simulink model "db4_8znzrb"  (R2018a)
settings: Solver=ode23s  StartTime=0.0  StopTime=0.45  MaxStep=1e-3  RelTol=1e-4  AbsTol=1e-3
values from neighbouring files (symbols this model uses):
  Ian = 5    [set_motor.m]
  Kn = 0.6    [set_motor.m]
libraries: simulink x2
settings Model: ExtModeTrigMode=oneshot  ExtModeArmWhenConnect=off  Creator=Lac User  LastModifiedBy=Matias
settings SolverCC: AutoScaleAbsTol=off  MaxOrder=1  ZeroCrossAlgorithm=Adaptive
settings DataIOCC: LimitDataPoints=on  SaveFormat=Array  SignalLoggingSaveFormat=ModelDataLogs  SaveOutput=off  SaveTime=off
settings OptimizationCC: BlockReduction=off  BooleanDataType=off  LifeSpan=inf
settings DebuggingCC: SaveWithParameterizedLinksMsg=none  UnderspecifiedInitializationDetection=Classic  MergeDetectMultiDrivingBlocksExec=none  SignalResolutionControl=TryResolveAllWithWarning  MultiTaskDSMMsg=warning  MultiTaskCondExecSysMsg=none  SFUnexpectedBacktrackingDiag=warning  SFNoUnconditionalDefaultTransitionDiag=warning  SFExecutionAtInitializationDiag=none
settings HardwareCC: ProdBitPerPointer=32  ProdBitPerSizeT=32  ProdBitPerPtrDiffT=32  ProdLargestAtomicFloat=None  ProdIntDivRoundTo=Undefined  ProdEndianess=Unspecified  ProdWordSize=32  ProdHWDeviceType=32-bit Generic  TargetUnknown=on
settings ModelReferenceCC: PropagateSignalLabelsOutOfModel=off
settings RTWCC: TemplateMakefile=grt_vc.tmf
settings CodeAppCC: StateflowObjectComments=on
settings GRTTargetCC: TargetLangStandard=C89/C90 (ANSI)  GeneratePreprocessorConditionals=Disable all  CombineOutputUpdateFcns=off  GRTInterface=on
settings ConfigComp: CovMetricSettings=dw  CovHtmlReporting=on  CovSaveCumulativeToWorkspaceVar=on  CovSaveSingleToWorkspaceVar=on  CovExternalEMLEnable=off

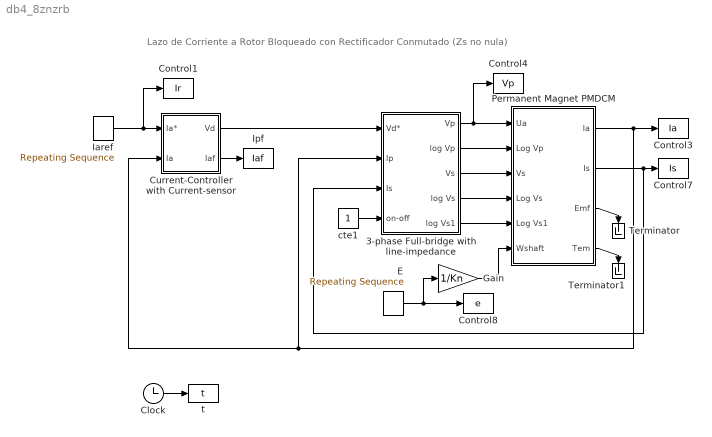
== system db4_8znzrb ==
  note: Lazo de Corriente a Rotor Bloqueado con Rectificador Conmutado (Zs no nula)
  3-phase Full-bridge with line-impedance : Subsystem  mask(3-phase Full-bridge with line-impedance){Vph=220, f=50, Rd=0.05, Ld=0.003, Rs=0.006, Ls=0.0002}
      mask prompts: Vph "RMS Phase Voltage [V]:"; f "Frecuency [Hz]:"; Rd "Armature Resistance [Ohms]:"; Ld "Armature Inductance  [Hy]:"; Rs "Line Resistance [Ohms]:"; Ls "Line Inductance [Hy]:"
  Clock : Clock
  Control1 : ToWorkspace  VariableName=Ir
      settings: MaxDataPoints=200000
  Control3 : ToWorkspace  VariableName=Ia
      settings: MaxDataPoints=200000
  Control4 : ToWorkspace  VariableName=Vp
      settings: MaxDataPoints=200000
  Control7 : ToWorkspace  VariableName=Is
      settings: MaxDataPoints=200000
  Control8 : ToWorkspace  VariableName=e
      settings: MaxDataPoints=200000
  Current-Controller with Current-sensor : Subsystem  mask(Current-Controller with Current-sensor){Kpi=0.16, TIi=0.027, Kti=1, Tfi=0.008, VLL=380}
      mask prompts: Kpi "Current Proportional Gain:"; TIi "Current Integral Gain:"; Kti "Current-sensor Proportional Gain:"; Tfi "Current-sensor Integral Gain:"; VLL "RMS Line to Line Voltage [V]:"
  E : simulink/Sources/Repeating Sequence  rep_seq_t="[0   0.4]"  rep_seq_y="[10   10 ]"
  Gain : Gain  Gain=1/Kn  SaturateOnIntegerOverflow=on  OutDataTypeStr=Inherit: Same as input  ParamDataTypeStr=Inherit: Same as input
  Iaref : simulink/Sources/Repeating Sequence  rep_seq_t=[0 0.4]  rep_seq_y=[Ian Ian]
  Ipf : ToWorkspace  VariableName=Iaf
      settings: MaxDataPoints=200000
  Permanent Magnet PMDCM : Subsystem  mask(Permanent Magnet PMDCM){La=0.003, Ra=0.05, k=6.7851, ic=0, Ls=0.0002, Rs=0.006}
      mask prompts: La "Armature Inductance  [Hy]:"; Ra "Armature Resistance [Ohms]:"; k "Motor Constant:"; ic "Armature Current Initial Condition [Amp]:"; Ls "Line Inductance [Hy]:"; Rs "Line Resistance [Ohms]:"
  Terminator : Terminator
  Terminator1 : Terminator
  cte1 : Constant
  t : ToWorkspace  VariableName=t
      settings: MaxDataPoints=200000
  wires:
  Iaref/1 -> Control1/1, Current-Controller with Current-sensor/1(Ia*)
  Current-Controller with Current-sensor/2(Iaf) -> Ipf/1
  E/1 -> Control8/1, Gain/1
  cte1/1 -> 3-phase Full-bridge with line-impedance/4(on-off)
  Current-Controller with Current-sensor/1(Vd) -> 3-phase Full-bridge with line-impedance/1(Vd*)
  3-phase Full-bridge with line-impedance/1(Vp) -> Control4/1, Permanent Magnet PMDCM/1(Ua)
  Gain/1 -> Permanent Magnet PMDCM/6(Wshaft)
  3-phase Full-bridge with line-impedance/2(log Vp) -> Permanent Magnet PMDCM/2(Log Vp)
  3-phase Full-bridge with line-impedance/3(Vs) -> Permanent Magnet PMDCM/3(Vs)
  3-phase Full-bridge with line-impedance/4(log Vs) -> Permanent Magnet PMDCM/4(Log Vs)
  3-phase Full-bridge with line-impedance/5(log Vs1) -> Permanent Magnet PMDCM/5(Log Vs1)
  Permanent Magnet PMDCM/1(Ia) -> Control3/1, Current-Controller with Current-sensor/2(Ia), 3-phase Full-bridge with line-impedance/2(Ip)
  Permanent Magnet PMDCM/2(Is) -> 3-phase Full-bridge with line-impedance/3(Is), Control7/1
  Permanent Magnet PMDCM/3(Emf) -> Terminator/1
  Permanent Magnet PMDCM/4(Tem) -> Terminator1/1
  Clock/1 -> t/1

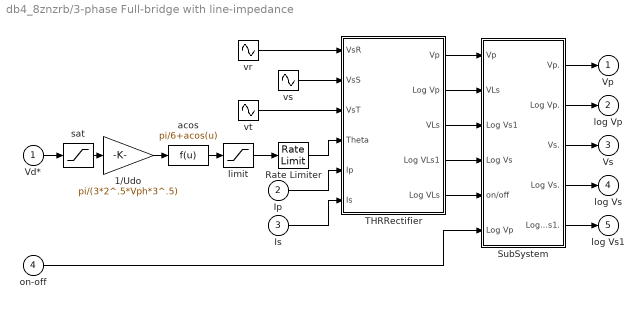
== system db4_8znzrb/3-phase Full-bridge with line-impedance ==
  Vd* : Inport
  Ip : Inport  Port=2
  Is : Inport  Port=3
  on-off : Inport  Port=4
  1/Udo : Gain  Gain=pi/(3*2^.5*Vph*3^.5)  SaturateOnIntegerOverflow=on  OutDataTypeStr=Inherit: Same as input  ParamDataTypeStr=Inherit: Same as input
  Rate Limiter : RateLimiter  RisingSlewLimit=8000  FallingSlewLimit=-8000
  SubSystem : Subsystem
  THRRectifier : Subsystem
      mask Display:
      | plot([0.3 0.7 0.5 0.3],[0.4 0.4 0.6 0.4])
      | plot([0.3 0.7 ],[0.6 0.6])
      | plot([0.5 0.5 ],[0.6 0.7])
      | plot([0.5 0.5 ],[0.3 0.4])
      | plot([0.35 0.5],[0.7 0.6])
      | plot([0.25 0.35 ],[0.7 0.7])
  acos : Fcn  Expr=pi/6+acos(u)
  limit : Saturate  UpperLimit=pi*6.999/6  LowerLimit=pi/5.998
  sat : Saturate  UpperLimit=(3*2^.5*3^.5*Vph)/pi  LowerLimit=-(3*2^.5*3^.5*Vph)/pi
  vr : Sin  Amplitude=Vph*(2^.5)  Frequency=2*f*pi  SampleTime=0
  vs : Sin  Amplitude=Vph*(2^.5)  Frequency=2*pi*f  Phase=-(2/3)*pi  SampleTime=0
  vt : Sin  Amplitude=Vph*(2^.5)  Frequency=2*pi*f  Phase=-(4/3)*pi  SampleTime=0
  Vp : Outport
  log Vp : Outport  Port=2
  Vs : Outport  Port=3
  log Vs : Outport  Port=4
  log Vs1 : Outport  Port=5
  wires:
  1/Udo/1 -> acos/1
  acos/1 -> limit/1
  vt/1 -> THRRectifier/3(VsT)
  vs/1 -> THRRectifier/2(VsS)
  vr/1 -> THRRectifier/1(VsR)
  Vd*/1 -> sat/1
  Ip/1 -> THRRectifier/5(Ip)
  Is/1 -> THRRectifier/6(Is)
  sat/1 -> 1/Udo/1
  limit/1 -> Rate Limiter/1
  THRRectifier/1(Vp) -> SubSystem/1(Vp)
  THRRectifier/2(Log Vp) -> SubSystem/2(VLs)
  THRRectifier/3(VLs) -> SubSystem/3(Log Vs1)
  THRRectifier/4(Log VLs1) -> SubSystem/4(Log Vs)
  THRRectifier/5(Log VLs) -> SubSystem/5(on/off)
  on-off/1 -> SubSystem/6(Log Vp)
  SubSystem/2(Log Vp.) -> log Vp/1
  SubSystem/3(Vs.) -> Vs/1
  SubSystem/4(Log Vs.) -> log Vs/1
  SubSystem/5(Log Vs1.) -> log Vs1/1
  SubSystem/1(Vp.) -> Vp/1
  Rate Limiter/1 -> THRRectifier/4(Theta)

== system db4_8znzrb/Current-Controller with Current-sensor ==
  Ia* : Inport
  Ia : Inport  Port=2
  Ftr : TransferFcn  Numerator=[Kti]  Denominator=[Tfi 1]
  I - Ctr : Subsystem
      mask Display: plot([0 .01  5],[0 2 4])
  Sum1 : Sum  Inputs=+-  SaturateOnIntegerOverflow=on  InputSameDT=on  OutDataTypeStr=Inherit: Same as first input
  Vd : Outport
  Iaf : Outport  Port=2
  wires:
  Ia*/1 -> Sum1/1
  Ia/1 -> Ftr/1, I - Ctr/2(Ia)
  Sum1/1 -> I - Ctr/1(Ia*- Iaf)
  I - Ctr/1(Vd*) -> Vd/1
  Ftr/1 -> Sum1/2, Iaf/1

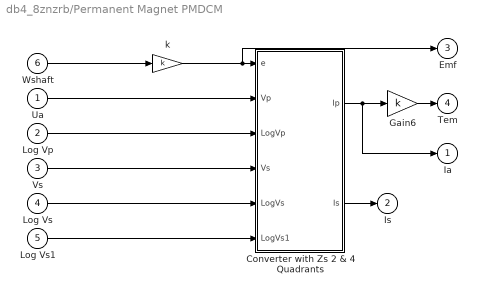
== system db4_8znzrb/Permanent Magnet PMDCM ==
  Ua : Inport
  Log Vp : Inport  Port=2
  Vs : Inport  Port=3
  Log Vs : Inport  Port=4
  Log Vs1 : Inport  Port=5
  Wshaft : Inport  Port=6
  Converter with Zs 2 & 4 Quadrants : Subsystem
  Gain6 : Gain  Gain=k  SaturateOnIntegerOverflow=on  OutDataTypeStr=Inherit: Same as input  ParamDataTypeStr=Inherit: Same as input
  k : Gain  Gain=k  SaturateOnIntegerOverflow=on  OutDataTypeStr=Inherit: Same as input  ParamDataTypeStr=Inherit: Same as input
  Ia : Outport
  Is : Outport  Port=2
  Emf : Outport  Port=3
  Tem : Outport  Port=4
  wires:
  k/1 -> Converter with Zs 2 & 4 Quadrants/1(e), Emf/1
  Ua/1 -> Converter with Zs 2 & 4 Quadrants/2(Vp)
  Log Vp/1 -> Converter with Zs 2 & 4 Quadrants/3(LogVp)
  Vs/1 -> Converter with Zs 2 & 4 Quadrants/4(Vs)
  Log Vs/1 -> Converter with Zs 2 & 4 Quadrants/5(LogVs)
  Log Vs1/1 -> Converter with Zs 2 & 4 Quadrants/6(LogVs1)
  Wshaft/1 -> k/1
  Converter with Zs 2 & 4 Quadrants/2(Is) -> Is/1
  Gain6/1 -> Tem/1
  Converter with Zs 2 & 4 Quadrants/1(Ip) -> Ia/1, Gain6/1

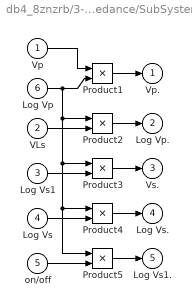
== system db4_8znzrb/3-phase Full-bridge with line-impedance/SubSystem ==
  Vp : Inport
  VLs : Inport  Port=2
  Log Vs1 : Inport  Port=3
  Log Vs : Inport  Port=4
  on/off : Inport  Port=5
  Log Vp : Inport  Port=6
  Product{1..5} (5 alike) : Product  SaturateOnIntegerOverflow=on  RndMeth=Zero  InputSameDT=on  OutDataTypeStr=Inherit: Same as first input
  Vp. : Outport
  Log Vp. : Outport  Port=2
  Vs. : Outport  Port=3
  Log Vs. : Outport  Port=4
  Log Vs1. : Outport  Port=5
  wires:
  VLs/1 -> Product2/2
  Log Vp/1 -> Product1/2, Product2/1, Product5/1, Product4/1, Product3/1
  Product2/1 -> Log Vp./1
  Product1/1 -> Vp./1
  Vp/1 -> Product1/1
  Log Vs1/1 -> Product3/2
  Log Vs/1 -> Product4/2
  on/off/1 -> Product5/2
  Product5/1 -> Log Vs1./1
  Product4/1 -> Log Vs./1
  Product3/1 -> Vs./1

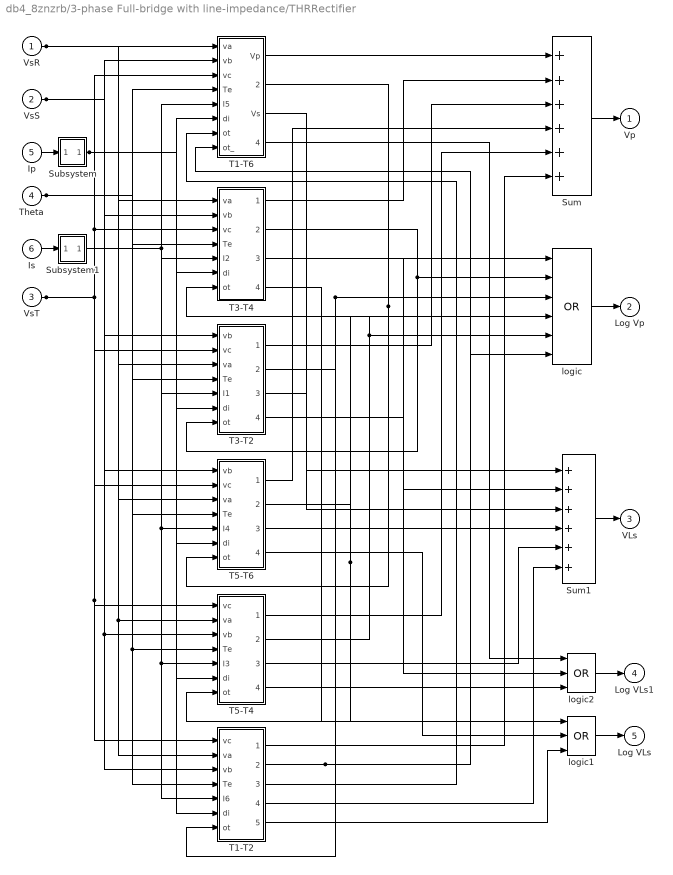
== system db4_8znzrb/3-phase Full-bridge with line-impedance/THRRectifier ==
  VsR : Inport
  VsS : Inport  Port=2
  VsT : Inport  Port=3
  Theta : Inport  Port=4
  Ip : Inport  Port=5
  Is : Inport  Port=6
  Subsystem : Subsystem
  Subsystem1 : Subsystem
  Sum : Sum  Inputs=++++++  SaturateOnIntegerOverflow=on  InputSameDT=on  OutDataTypeStr=Inherit: Same as first input
  Sum1 : Sum  Inputs=++++++  SaturateOnIntegerOverflow=on  InputSameDT=on  OutDataTypeStr=Inherit: Same as first input
  T1-T2 : Subsystem
  T1-T6 : Subsystem
  T3-T2 : Subsystem
  T3-T4 : Subsystem
  T5-T4 : Subsystem
  T5-T6 : Subsystem
  logic : Logic  Operator=OR  Inputs=6
  logic1 : Logic  Operator=OR  Inputs=3
  logic2 : Logic  Operator=OR  Inputs=3
  Vp : Outport
  Log Vp : Outport  Port=2
  VLs : Outport  Port=3
  Log VLs1 : Outport  Port=4
  Log VLs : Outport  Port=5
  wires:
  logic2/1 -> Log VLs1/1
  logic1/1 -> Log VLs/1
  Subsystem1/1(out_1) -> T1-T6/5(I5), T1-T2/5(I6), T5-T4/5(I3), T5-T6/5(I4), T3-T4/5(I2), T3-T2/5(I1)
  Subsystem/1(out_1) -> T5-T4/6(di), T5-T6/6(di), T3-T2/6(di), T3-T4/6(di), T1-T6/6(di), T1-T2/6(di)
  Theta/1 -> T1-T2/4(Te), T5-T4/4(Te), T5-T6/4(Te), T3-T2/4(Te), T3-T4/4(Te), T1-T6/4(Te)
  T1-T2/2(out_1) -> T1-T6/8(ot_), logic/6
  logic/1 -> Log Vp/1
  Sum/1 -> Vp/1
  Ip/1 -> Subsystem/1(in_1)
  Sum1/1 -> VLs/1
  T1-T6/2(Log Vp) -> T5-T6/7(ot), logic/1
  T1-T6/1(Vp) -> Sum/1
  T1-T6/3(Vs) -> Sum1/1
  T1-T6/4(Log Vs) -> logic2/1
  T3-T4/1(out_2) -> Sum/2
  VsR/1 -> T1-T6/1(va), T3-T4/1(va), T3-T2/3(va), T5-T6/3(va), T5-T4/2(va), T1-T2/2(va)
  VsS/1 -> T1-T6/2(vb), T3-T4/2(vb), T3-T2/1(vb), T5-T6/1(vb), T5-T4/3(vb), T1-T2/3(vb)
  T3-T4/2(out_1) -> T3-T2/7(ot), logic/2
  T3-T4/3(out_3) -> Sum1/2
  T3-T4/4(out_4) -> logic1/1
  T3-T2/1(out_2) -> Sum/3
  T3-T2/2(out_1) -> logic/3, T1-T2/7(ot)
  T3-T2/3(out_3) -> Sum1/3
  T3-T2/4(out_4) -> logic2/2
  VsT/1 -> T3-T2/2(vc), T1-T6/3(vc), T3-T4/3(vc), T5-T6/2(vc), T5-T4/1(vc), T1-T2/1(vc)
  T5-T6/2(out_1) -> T5-T4/7(ot), logic/4
  T5-T6/3(out_3) -> Sum1/4
  T5-T6/4(out_4) -> logic1/2
  T5-T6/1(out_2) -> Sum/4
  T5-T4/2(out_1) -> T3-T4/7(ot), logic/5
  T5-T4/1(out_2) -> Sum/5
  T5-T4/3(out_3) -> Sum1/5
  T5-T4/4(out_4) -> logic2/3
  T1-T2/3(out_3) -> T1-T6/7(ot)
  T1-T2/4("out_4 ") -> Sum1/6
  T1-T2/5(out_5) -> logic1/3
  T1-T2/1(out_2) -> Sum/6
  Is/1 -> Subsystem1/1(in_1)

== system db4_8znzrb/Current-Controller with Current-sensor/I - Ctr ==
  Ia*- Iaf : Inport
  Ia : Inport  Port=2
  Adaptative Control : Subsystem
  comp : RelationalOperator  Operator=>  RndMeth=Nearest  InputSameDT=on
  cte1 : Constant  Value=0
  sat : Saturate  UpperLimit=VLL*sqrt(2)*3/pi  LowerLimit=-VLL*sqrt(2)*3/pi
  Vd* : Outport
  wires:
  Ia*- Iaf/1 -> Adaptative Control/2(Ia*- Iaf)
  cte1/1 -> comp/2
  sat/1 -> Vd*/1
  Adaptative Control/1(Vd*) -> sat/1
  comp/1 -> Adaptative Control/1(Ia>0)
  Ia/1 -> comp/1

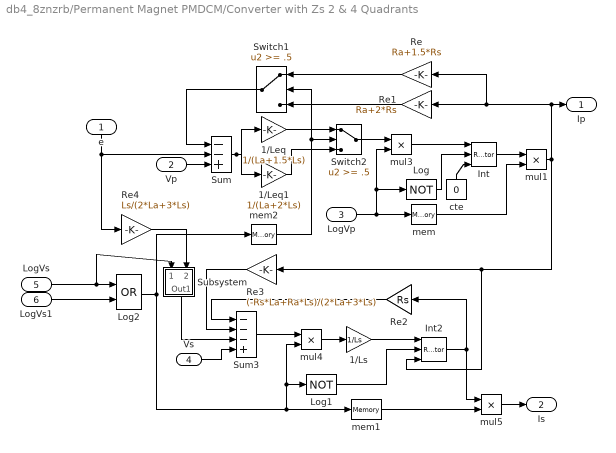
== system db4_8znzrb/Permanent Magnet PMDCM/Converter with Zs 2 & 4 Quadrants ==
  e : Inport
  Vp : Inport  Port=2
  LogVp : Inport  Port=3
  Vs : Inport  Port=4
  LogVs : Inport  Port=5
  LogVs1 : Inport  Port=6
  "1/Leq " : Gain  Gain=1/(La+1.5*Ls)  SaturateOnIntegerOverflow=on  OutDataTypeStr=Inherit: Same as input  ParamDataTypeStr=Inherit: Same as input
  1/Leq1 : Gain  Gain=1/(La+2*Ls)  SaturateOnIntegerOverflow=on  OutDataTypeStr=Inherit: Same as input  ParamDataTypeStr=Inherit: Same as input
  1/Ls : Gain  Gain=1/Ls  SaturateOnIntegerOverflow=on  OutDataTypeStr=Inherit: Same as input  ParamDataTypeStr=Inherit: Same as input
  Int : ResetIntegrator
  Int2 : ResetIntegrator
  Log : Logic  Operator=NOT  Inputs=1
  Log1 : Logic  Operator=NOT  Inputs=1
  Log2 : Logic  Operator=OR
  Re : Gain  Gain=Ra+1.5*Rs  SaturateOnIntegerOverflow=on  OutDataTypeStr=Inherit: Same as input  ParamDataTypeStr=Inherit: Same as input
  Re1 : Gain  Gain=Ra+2*Rs  SaturateOnIntegerOverflow=on  OutDataTypeStr=Inherit: Same as input  ParamDataTypeStr=Inherit: Same as input
  Re2 : Gain  Gain=Rs  SaturateOnIntegerOverflow=on  OutDataTypeStr=Inherit: Same as input  ParamDataTypeStr=Inherit: Same as input
  Re3 : Gain  Gain=(-Rs*La+Ra*Ls)/(2*La+3*Ls)  SaturateOnIntegerOverflow=on  OutDataTypeStr=Inherit: Same as input  ParamDataTypeStr=Inherit: Same as input
  Re4 : Gain  Gain=Ls/(2*La+3*Ls)  SaturateOnIntegerOverflow=on  OutDataTypeStr=Inherit: Same as input  ParamDataTypeStr=Inherit: Same as input
  Subsystem : Subsystem
      mask Display: disp('-1')
  Sum : Sum  Inputs=--+  SaturateOnIntegerOverflow=on  InputSameDT=on  OutDataTypeStr=Inherit: Same as first input
  Sum3 : Sum  Inputs=---+  SaturateOnIntegerOverflow=on  InputSameDT=on  OutDataTypeStr=Inherit: Same as first input
  Switch1 : Switch  Threshold=.5  SaturateOnIntegerOverflow=on  InputSameDT=on
  Switch2 : Switch  Threshold=.5  SaturateOnIntegerOverflow=on  InputSameDT=on
  cte : Constant  Value=0
  mem : Memory
  mem1 : Memory
  mem2 : Memory
  mul{1,3..5} (4 alike) : Product  SaturateOnIntegerOverflow=on  RndMeth=Zero  InputSameDT=on  OutDataTypeStr=Inherit: Same as first input
  Ip : Outport
  Is : Outport  Port=2
  wires:
  mem/1 -> mul1/2
  Int/1 -> mul1/1
  mul3/1 -> Int/1
  Log/1 -> Int/2
  cte/1 -> Int/3
  mul1/1 -> Re3/1, Int2/3, Ip/1, Re1/1, Re/1
  LogVp/1 -> mem/1, mul3/2, Log/1
  Switch2/1 -> mul3/1
  1/Leq1/1 -> Switch2/3
  "1/Leq "/1 -> Switch2/1
  Re/1 -> Switch1/1
  Re1/1 -> Switch1/3
  Vp/1 -> Sum/3
  mem2/1 -> Switch1/2, Switch2/2
  Sum/1 -> 1/Leq1/1, "1/Leq "/1
  Re3/1 -> Sum3/2
  Switch1/1 -> Sum/1
  LogVs/1 -> Subsystem/1(In1), Log2/1
  Vs/1 -> Sum3/4
  mul5/1 -> Is/1
  Re4/1 -> Subsystem/2(In2)
  Log2/1 -> mem2/1, mul4/2, Log1/1, mem1/1
  1/Ls/1 -> Int2/1
  mul4/1 -> 1/Ls/1
  Log1/1 -> Int2/2
  Re2/1 -> Sum3/1
  Sum3/1 -> mul4/1
  mem1/1 -> mul5/2
  Int2/1 -> Re2/1, mul5/1
  e/1 -> Sum/2, Re4/1
  Subsystem/1(Out1) -> Sum3/3
  LogVs1/1 -> Log2/2

== system db4_8znzrb/3-phase Full-bridge with line-impedance/THRRectifier/Subsystem ==
  in_1 : Inport
  comp : RelationalOperator  Operator=>  RndMeth=Nearest  InputSameDT=on
  cte : Constant  Value=0
  out_1 : Outport
  wires:
  cte/1 -> comp/2
  in_1/1 -> comp/1
  comp/1 -> out_1/1

== system db4_8znzrb/3-phase Full-bridge with line-impedance/THRRectifier/Subsystem1 ==
  in_1 : Inport
  Vdset : Step  Time=0  Before=1  SampleTime=0
  comp : RelationalOperator  Operator=>  RndMeth=Nearest  InputSameDT=on
  cte : Constant  Value=0
  mul : Product  SaturateOnIntegerOverflow=on  RndMeth=Zero  InputSameDT=on  OutDataTypeStr=Inherit: Same as first input
  out_1 : Outport
  wires:
  Vdset/1 -> mul/2
  mul/1 -> out_1/1
  comp/1 -> mul/1
  cte/1 -> comp/2
  in_1/1 -> comp/1

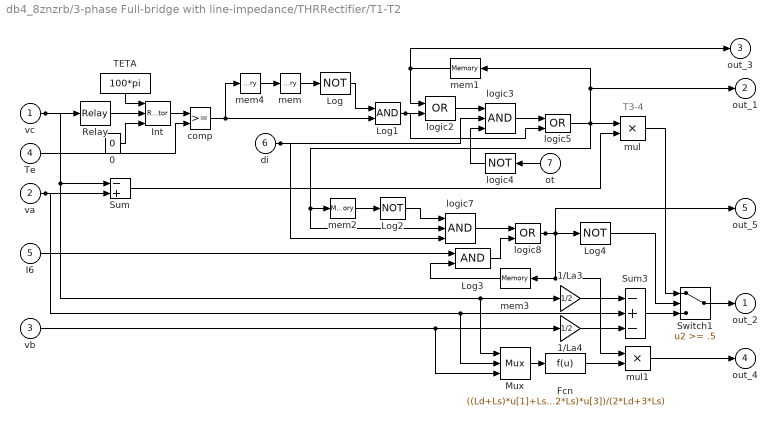
== system db4_8znzrb/3-phase Full-bridge with line-impedance/THRRectifier/T1-T2 ==
  note: T3-4
  vc : Inport
  va : Inport  Port=2
  vb : Inport  Port=3
  Te : Inport  Port=4
  I6 : Inport  Port=5
  di : Inport  Port=6
  ot : Inport  Port=7
  0 : Constant  Value=0
  1/La3 : Gain  Gain=1/2  SaturateOnIntegerOverflow=on  OutDataTypeStr=Inherit: Same as input  ParamDataTypeStr=Inherit: Same as input
  1/La4 : Gain  Gain=1/2  SaturateOnIntegerOverflow=on  OutDataTypeStr=Inherit: Same as input  ParamDataTypeStr=Inherit: Same as input
  Fcn : Fcn  Expr=((Ld+Ls)*u[1]+Ls*u[2]-(Ld+2*Ls)*u[3])/(2*Ld+3*Ls)
  Int : ResetIntegrator
  Log : Logic  Operator=NOT  Inputs=1
  Log1 : Logic
  Log2 : Logic  Operator=NOT  Inputs=1
  Log3 : Logic
  Log4 : Logic  Operator=NOT  Inputs=1
  Mux : Mux  Inputs=3
  Relay : Relay  OnSwitchValue=(2^.5)*Vph*sin(pi/6)  OffSwitchValue=0
  Sum : Sum  Inputs=-+  SaturateOnIntegerOverflow=on  InputSameDT=on  OutDataTypeStr=Inherit: Same as first input
  Sum3 : Sum  Inputs=-+-  SaturateOnIntegerOverflow=on  InputSameDT=on  OutDataTypeStr=Inherit: Same as first input
  Switch1 : Switch  Threshold=.5  SaturateOnIntegerOverflow=on  InputSameDT=on
  TETA : Constant  Value=100*pi
  comp : RelationalOperator  RndMeth=Nearest  InputSameDT=on
  logic2 : Logic  Operator=OR
  logic3 : Logic  Inputs=3
  logic4 : Logic  Operator=NOT  Inputs=1
  logic5 : Logic  Operator=OR
  logic7 : Logic  Inputs=3
  logic8 : Logic  Operator=OR
  mem{,1..4} (5 alike) : Memory
  mul : Product  SaturateOnIntegerOverflow=on  RndMeth=Zero  InputSameDT=on  OutDataTypeStr=Inherit: Same as first input
  mul1 : Product  SaturateOnIntegerOverflow=on  RndMeth=Zero  InputSameDT=on  OutDataTypeStr=Inherit: Same as first input
  out_2 : Outport
  out_1 : Outport  Port=2
  out_3 : Outport  Port=3
  "out_4 " : Outport  Port=4
  out_5 : Outport  Port=5
  wires:
  comp/1 -> Log1/2, mem4/1
  mem4/1 -> mem/1
  mem/1 -> Log/1
  logic4/1 -> logic3/3
  0/1 -> Int/3
  logic2/1 -> logic3/1
  TETA/1 -> Int/1
  Int/1 -> comp/1
  Te/1 -> comp/2
  ot/1 -> logic4/1
  Relay/1 -> Int/2
  logic3/1 -> logic5/1
  Log1/1 -> logic2/2, logic5/2
  logic5/1 -> mul/1, mem2/1, logic7/2, mem1/1, out_1/1
  mem2/1 -> Log2/1
  Log/1 -> Log1/1
  Log3/1 -> logic8/2
  logic7/1 -> logic8/1
  di/1 -> logic3/2, logic7/3
  Log2/1 -> logic7/1
  1/La4/1 -> Sum3/3
  1/La3/1 -> Sum3/1
  Sum3/1 -> Switch1/3
  mul/1 -> Switch1/1
  mem3/1 -> Log3/2
  Log4/1 -> Switch1/2
  Switch1/1 -> out_2/1
  I6/1 -> Log3/1
  Sum/1 -> mul/2
  mem1/1 -> logic2/1, out_3/1
  Mux/1 -> Fcn/1
  vc/1 -> Relay/1, Sum/1, 1/La3/1, Mux/1
  va/1 -> Sum/2, Sum3/2, Mux/2
  vb/1 -> 1/La4/1, Mux/3
  mul1/1 -> "out_4 "/1
  Fcn/1 -> mul1/2
  logic8/1 -> out_5/1, Log4/1, mem3/1, mul1/1

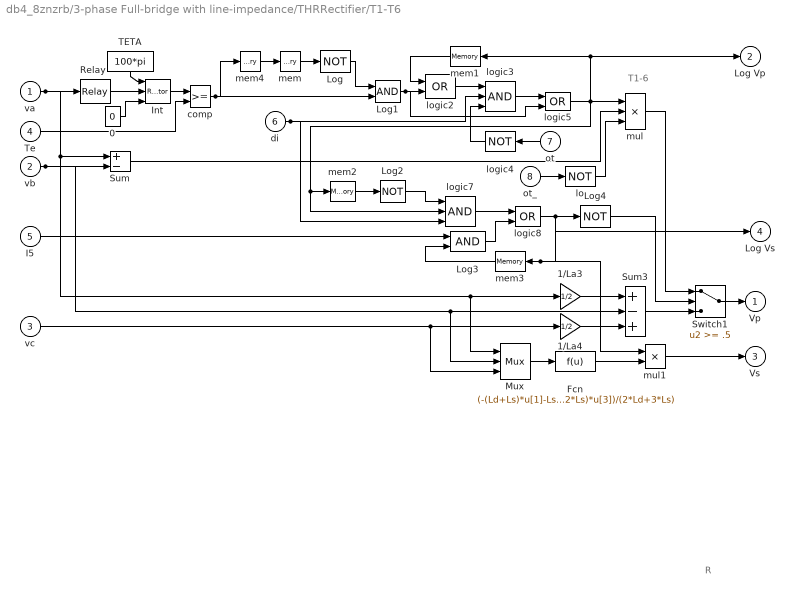
== system db4_8znzrb/3-phase Full-bridge with line-impedance/THRRectifier/T1-T6 ==
  note: R
  note: T1-6
  va : Inport
  vb : Inport  Port=2
  vc : Inport  Port=3
  Te : Inport  Port=4
  I5 : Inport  Port=5
  di : Inport  Port=6
  ot : Inport  Port=7
  ot_ : Inport  Port=8
  0 : Constant  Value=0
  1/La3 : Gain  Gain=1/2  SaturateOnIntegerOverflow=on  OutDataTypeStr=Inherit: Same as input  ParamDataTypeStr=Inherit: Same as input
  1/La4 : Gain  Gain=1/2  SaturateOnIntegerOverflow=on  OutDataTypeStr=Inherit: Same as input  ParamDataTypeStr=Inherit: Same as input
  Fcn : Fcn  Expr=(-(Ld+Ls)*u[1]-Ls*u[2]+(Ld+2*Ls)*u[3])/(2*Ld+3*Ls)
  Int : ResetIntegrator
  Log : Logic  Operator=NOT  Inputs=1
  Log1 : Logic
  Log2 : Logic  Operator=NOT  Inputs=1
  Log3 : Logic
  Log4 : Logic  Operator=NOT  Inputs=1
  Mux : Mux  Inputs=3
  Relay : Relay  OnSwitchValue=0  OffSwitchValue=(2^.5)*Vph*sin(pi/6+pi)  OnOutputValue=0  OffOutputValue=1
  Sum : Sum  Inputs=+-  SaturateOnIntegerOverflow=on  InputSameDT=on  OutDataTypeStr=Inherit: Same as first input
  Sum3 : Sum  Inputs=+-+  SaturateOnIntegerOverflow=on  InputSameDT=on  OutDataTypeStr=Inherit: Same as first input
  Switch1 : Switch  Threshold=.5  SaturateOnIntegerOverflow=on  InputSameDT=on
  TETA : Constant  Value=100*pi
  comp : RelationalOperator  RndMeth=Nearest  InputSameDT=on
  lo : Logic  Operator=NOT  Inputs=1
  logic2 : Logic  Operator=OR
  logic3 : Logic  Inputs=3
  logic4 : Logic  Operator=NOT  Inputs=1
  logic5 : Logic  Operator=OR
  logic7 : Logic  Inputs=3
  logic8 : Logic  Operator=OR
  mem{,1..4} (5 alike) : Memory
  mul : Product  Inputs=3  SaturateOnIntegerOverflow=on  RndMeth=Zero  InputSameDT=on  OutDataTypeStr=Inherit: Same as first input
  mul1 : Product  SaturateOnIntegerOverflow=on  RndMeth=Zero  InputSameDT=on  OutDataTypeStr=Inherit: Same as first input
  Vp : Outport
  Log Vp : Outport  Port=2
  Vs : Outport  Port=3
  Log Vs : Outport  Port=4
  wires:
  logic8/1 -> mem3/1, mul1/1, Log4/1, Log Vs/1
  di/1 -> logic7/3, logic3/2
  comp/1 -> Log1/2, mem4/1
  mem4/1 -> mem/1
  lo/1 -> mul/3
  logic4/1 -> logic3/3
  mem1/1 -> logic2/1
  mem/1 -> Log/1
  0/1 -> Int/3
  logic2/1 -> logic3/1
  TETA/1 -> Int/1
  Int/1 -> comp/1
  Te/1 -> comp/2
  ot/1 -> logic4/1
  ot_/1 -> lo/1
  Relay/1 -> Int/2
  logic3/1 -> logic5/1
  Log1/1 -> logic2/2, logic5/2
  logic5/1 -> mul/1, Log Vp/1, mem1/1, mem2/1, logic7/2
  mem2/1 -> Log2/1
  Log/1 -> Log1/1
  Log3/1 -> logic8/2
  logic7/1 -> logic8/1
  Log2/1 -> logic7/1
  1/La4/1 -> Sum3/3
  1/La3/1 -> Sum3/1
  Sum3/1 -> Switch1/3
  mul/1 -> Switch1/1
  mem3/1 -> Log3/2
  Log4/1 -> Switch1/2
  Switch1/1 -> Vp/1
  I5/1 -> Log3/1
  Sum/1 -> mul/2
  Mux/1 -> Fcn/1
  va/1 -> Relay/1, Sum/1, 1/La3/1, Mux/1
  vb/1 -> Sum/2, Sum3/2, Mux/2
  vc/1 -> 1/La4/1, Mux/3
  Fcn/1 -> mul1/2
  mul1/1 -> Vs/1

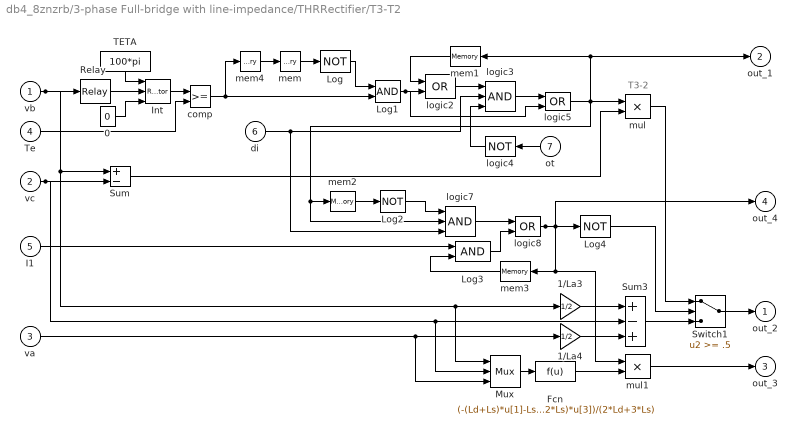
== system db4_8znzrb/3-phase Full-bridge with line-impedance/THRRectifier/T3-T2 ==
  note: T3-2
  vb : Inport
  vc : Inport  Port=2
  va : Inport  Port=3
  Te : Inport  Port=4
  I1 : Inport  Port=5
  di : Inport  Port=6
  ot : Inport  Port=7
  0 : Constant  Value=0
  1/La3 : Gain  Gain=1/2  SaturateOnIntegerOverflow=on  OutDataTypeStr=Inherit: Same as input  ParamDataTypeStr=Inherit: Same as input
  1/La4 : Gain  Gain=1/2  SaturateOnIntegerOverflow=on  OutDataTypeStr=Inherit: Same as input  ParamDataTypeStr=Inherit: Same as input
  Fcn : Fcn  Expr=(-(Ld+Ls)*u[1]-Ls*u[2]+(Ld+2*Ls)*u[3])/(2*Ld+3*Ls)
  Int : ResetIntegrator
  Log : Logic  Operator=NOT  Inputs=1
  Log1 : Logic
  Log2 : Logic  Operator=NOT  Inputs=1
  Log3 : Logic
  Log4 : Logic  Operator=NOT  Inputs=1
  Mux : Mux  Inputs=3
  Relay : Relay  OnSwitchValue=0  OffSwitchValue=(2^.5)*Vph*sin(pi/6+pi)  OnOutputValue=0  OffOutputValue=1
  Sum : Sum  Inputs=+-  SaturateOnIntegerOverflow=on  InputSameDT=on  OutDataTypeStr=Inherit: Same as first input
  Sum3 : Sum  Inputs=+-+  SaturateOnIntegerOverflow=on  InputSameDT=on  OutDataTypeStr=Inherit: Same as first input
  Switch1 : Switch  Threshold=.5  SaturateOnIntegerOverflow=on  InputSameDT=on
  TETA : Constant  Value=100*pi
  comp : RelationalOperator  RndMeth=Nearest  InputSameDT=on
  logic2 : Logic  Operator=OR
  logic3 : Logic  Inputs=3
  logic4 : Logic  Operator=NOT  Inputs=1
  logic5 : Logic  Operator=OR
  logic7 : Logic  Inputs=3
  logic8 : Logic  Operator=OR
  mem{,1..4} (5 alike) : Memory
  mul : Product  SaturateOnIntegerOverflow=on  RndMeth=Zero  InputSameDT=on  OutDataTypeStr=Inherit: Same as first input
  mul1 : Product  SaturateOnIntegerOverflow=on  RndMeth=Zero  InputSameDT=on  OutDataTypeStr=Inherit: Same as first input
  out_2 : Outport
  out_1 : Outport  Port=2
  out_3 : Outport  Port=3
  out_4 : Outport  Port=4
  wires:
  comp/1 -> Log1/2, mem4/1
  di/1 -> logic3/2, logic7/3
  mem4/1 -> mem/1
  mem/1 -> Log/1
  Sum/1 -> mul/2
  I1/1 -> Log3/1
  Switch1/1 -> out_2/1
  Log4/1 -> Switch1/2
  logic8/1 -> out_4/1, Log4/1, mem3/1, mul1/1
  mem3/1 -> Log3/2
  mul/1 -> Switch1/1
  Sum3/1 -> Switch1/3
  1/La3/1 -> Sum3/1
  1/La4/1 -> Sum3/3
  logic5/1 -> mul/1, mem2/1, logic7/2, out_1/1, mem1/1
  Log2/1 -> logic7/1
  logic7/1 -> logic8/1
  Log3/1 -> logic8/2
  Log/1 -> Log1/1
  mem2/1 -> Log2/1
  logic3/1 -> logic5/1
  Relay/1 -> Int/2
  ot/1 -> logic4/1
  Te/1 -> comp/2
  Int/1 -> comp/1
  TETA/1 -> Int/1
  logic2/1 -> logic3/1
  0/1 -> Int/3
  Log1/1 -> logic5/2, logic2/2
  mem1/1 -> logic2/1
  logic4/1 -> logic3/3
  Mux/1 -> Fcn/1
  Fcn/1 -> mul1/2
  mul1/1 -> out_3/1
  vb/1 -> Relay/1, Sum/1, 1/La3/1, Mux/1
  vc/1 -> Sum/2, Sum3/2, Mux/2
  va/1 -> 1/La4/1, Mux/3

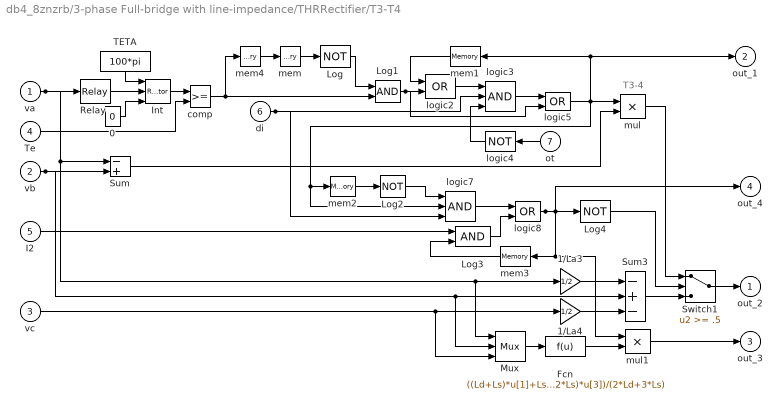
== system db4_8znzrb/3-phase Full-bridge with line-impedance/THRRectifier/T3-T4 ==
  note: T3-4
  va : Inport
  vb : Inport  Port=2
  vc : Inport  Port=3
  Te : Inport  Port=4
  I2 : Inport  Port=5
  di : Inport  Port=6
  ot : Inport  Port=7
  0 : Constant  Value=0
  1/La3 : Gain  Gain=1/2  SaturateOnIntegerOverflow=on  OutDataTypeStr=Inherit: Same as input  ParamDataTypeStr=Inherit: Same as input
  1/La4 : Gain  Gain=1/2  SaturateOnIntegerOverflow=on  OutDataTypeStr=Inherit: Same as input  ParamDataTypeStr=Inherit: Same as input
  Fcn : Fcn  Expr=((Ld+Ls)*u[1]+Ls*u[2]-(Ld+2*Ls)*u[3])/(2*Ld+3*Ls)
  Int : ResetIntegrator  InitialCondition=-1
  Log : Logic  Operator=NOT  Inputs=1
  Log1 : Logic
  Log2 : Logic  Operator=NOT  Inputs=1
  Log3 : Logic
  Log4 : Logic  Operator=NOT  Inputs=1
  Mux : Mux  Inputs=3
  Relay : Relay  OnSwitchValue=(2^.5)*Vph*sin(pi/6)  OffSwitchValue=0
  Sum : Sum  Inputs=-+  SaturateOnIntegerOverflow=on  InputSameDT=on  OutDataTypeStr=Inherit: Same as first input
  Sum3 : Sum  Inputs=-+-  SaturateOnIntegerOverflow=on  InputSameDT=on  OutDataTypeStr=Inherit: Same as first input
  Switch1 : Switch  Threshold=.5  SaturateOnIntegerOverflow=on  InputSameDT=on
  TETA : Constant  Value=100*pi
  comp : RelationalOperator  RndMeth=Nearest  InputSameDT=on
  logic2 : Logic  Operator=OR
  logic3 : Logic  Inputs=3
  logic4 : Logic  Operator=NOT  Inputs=1
  logic5 : Logic  Operator=OR
  logic7 : Logic  Inputs=3
  logic8 : Logic  Operator=OR
  mem{,1..4} (5 alike) : Memory
  mul : Product  SaturateOnIntegerOverflow=on  RndMeth=Zero  InputSameDT=on  OutDataTypeStr=Inherit: Same as first input
  mul1 : Product  SaturateOnIntegerOverflow=on  RndMeth=Zero  InputSameDT=on  OutDataTypeStr=Inherit: Same as first input
  out_2 : Outport
  out_1 : Outport  Port=2
  out_3 : Outport  Port=3
  out_4 : Outport  Port=4
  wires:
  comp/1 -> Log1/2, mem4/1
  mem4/1 -> mem/1
  mem/1 -> Log/1
  Sum/1 -> mul/2
  I2/1 -> Log3/1
  Switch1/1 -> out_2/1
  Log4/1 -> Switch1/2
  logic8/1 -> out_4/1, Log4/1, mem3/1, mul1/1
  mem3/1 -> Log3/2
  mul/1 -> Switch1/1
  Sum3/1 -> Switch1/3
  1/La3/1 -> Sum3/1
  1/La4/1 -> Sum3/3
  logic5/1 -> mul/1, mem2/1, logic7/2, out_1/1, mem1/1
  Log2/1 -> logic7/1
  di/1 -> logic3/2, logic7/3
  logic7/1 -> logic8/1
  Log3/1 -> logic8/2
  Log/1 -> Log1/1
  mem2/1 -> Log2/1
  logic3/1 -> logic5/1
  Relay/1 -> Int/2
  ot/1 -> logic4/1
  Te/1 -> comp/2
  Int/1 -> comp/1
  TETA/1 -> Int/1
  logic2/1 -> logic3/1
  0/1 -> Int/3
  Log1/1 -> logic5/2, logic2/2
  mem1/1 -> logic2/1
  logic4/1 -> logic3/3
  Mux/1 -> Fcn/1
  Fcn/1 -> mul1/2
  mul1/1 -> out_3/1
  va/1 -> Relay/1, Sum/1, 1/La3/1, Mux/1
  vb/1 -> Sum/2, Sum3/2, Mux/2
  vc/1 -> 1/La4/1, Mux/3

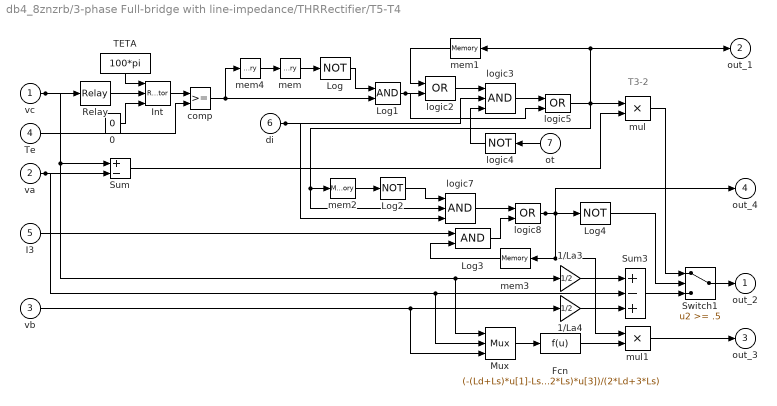
== system db4_8znzrb/3-phase Full-bridge with line-impedance/THRRectifier/T5-T4 ==
  note: T3-2
  vc : Inport
  va : Inport  Port=2
  vb : Inport  Port=3
  Te : Inport  Port=4
  I3 : Inport  Port=5
  di : Inport  Port=6
  ot : Inport  Port=7
  0 : Constant  Value=0
  1/La3 : Gain  Gain=1/2  SaturateOnIntegerOverflow=on  OutDataTypeStr=Inherit: Same as input  ParamDataTypeStr=Inherit: Same as input
  1/La4 : Gain  Gain=1/2  SaturateOnIntegerOverflow=on  OutDataTypeStr=Inherit: Same as input  ParamDataTypeStr=Inherit: Same as input
  Fcn : Fcn  Expr=(-(Ld+Ls)*u[1]-Ls*u[2]+(Ld+2*Ls)*u[3])/(2*Ld+3*Ls)
  Int : ResetIntegrator  InitialCondition=2/3*pi
  Log : Logic  Operator=NOT  Inputs=1
  Log1 : Logic
  Log2 : Logic  Operator=NOT  Inputs=1
  Log3 : Logic
  Log4 : Logic  Operator=NOT  Inputs=1
  Mux : Mux  Inputs=3
  Relay : Relay  OnSwitchValue=0  OffSwitchValue=(2^.5)*Vph*sin(pi/6+pi)  OnOutputValue=0  OffOutputValue=1
  Sum : Sum  Inputs=+-  SaturateOnIntegerOverflow=on  InputSameDT=on  OutDataTypeStr=Inherit: Same as first input
  Sum3 : Sum  Inputs=+-+  SaturateOnIntegerOverflow=on  InputSameDT=on  OutDataTypeStr=Inherit: Same as first input
  Switch1 : Switch  Threshold=.5  SaturateOnIntegerOverflow=on  InputSameDT=on
  TETA : Constant  Value=100*pi
  comp : RelationalOperator  RndMeth=Nearest  InputSameDT=on
  logic2 : Logic  Operator=OR
  logic3 : Logic  Inputs=3
  logic4 : Logic  Operator=NOT  Inputs=1
  logic5 : Logic  Operator=OR
  logic7 : Logic  Inputs=3
  logic8 : Logic  Operator=OR
  mem{,1..4} (5 alike) : Memory
  mul : Product  SaturateOnIntegerOverflow=on  RndMeth=Zero  InputSameDT=on  OutDataTypeStr=Inherit: Same as first input
  mul1 : Product  SaturateOnIntegerOverflow=on  RndMeth=Zero  InputSameDT=on  OutDataTypeStr=Inherit: Same as first input
  out_2 : Outport
  out_1 : Outport  Port=2
  out_3 : Outport  Port=3
  out_4 : Outport  Port=4
  wires:
  comp/1 -> Log1/2, mem4/1
  mem4/1 -> mem/1
  mem/1 -> Log/1
  logic4/1 -> logic3/3
  mem1/1 -> logic2/1
  0/1 -> Int/3
  logic2/1 -> logic3/1
  TETA/1 -> Int/1
  Int/1 -> comp/1
  di/1 -> logic7/3, logic3/2
  Te/1 -> comp/2
  ot/1 -> logic4/1
  Relay/1 -> Int/2
  logic3/1 -> logic5/1
  Log1/1 -> logic2/2, logic5/2
  logic5/1 -> mul/1, out_1/1, mem1/1, mem2/1, logic7/2
  mem2/1 -> Log2/1
  Log/1 -> Log1/1
  Log3/1 -> logic8/2
  logic7/1 -> logic8/1
  Log2/1 -> logic7/1
  1/La4/1 -> Sum3/3
  1/La3/1 -> Sum3/1
  Sum3/1 -> Switch1/3
  mul/1 -> Switch1/1
  mem3/1 -> Log3/2
  Log4/1 -> Switch1/2
  Switch1/1 -> out_2/1
  I3/1 -> Log3/1
  Sum/1 -> mul/2
  Mux/1 -> Fcn/1
  vc/1 -> Relay/1, Sum/1, 1/La3/1, Mux/1
  va/1 -> Sum/2, Sum3/2, Mux/2
  vb/1 -> 1/La4/1, Mux/3
  Fcn/1 -> mul1/2
  mul1/1 -> out_3/1
  logic8/1 -> out_4/1, Log4/1, mem3/1, mul1/1

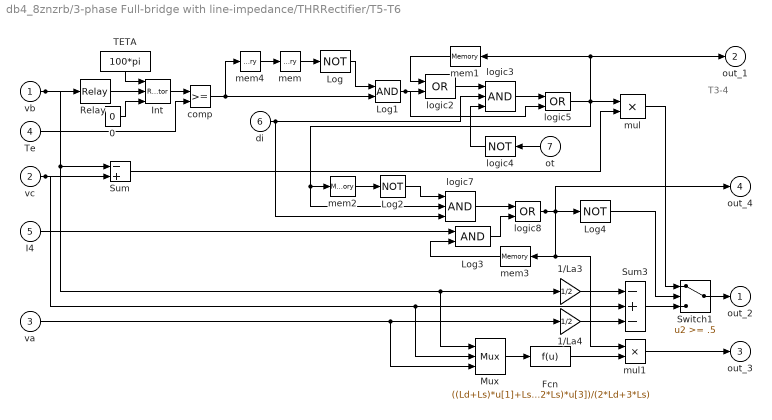
== system db4_8znzrb/3-phase Full-bridge with line-impedance/THRRectifier/T5-T6 ==
  note: T3-4
  vb : Inport
  vc : Inport  Port=2
  va : Inport  Port=3
  Te : Inport  Port=4
  I4 : Inport  Port=5
  di : Inport  Port=6
  ot : Inport  Port=7
  0 : Constant  Value=0
  1/La3 : Gain  Gain=1/2  SaturateOnIntegerOverflow=on  OutDataTypeStr=Inherit: Same as input  ParamDataTypeStr=Inherit: Same as input
  1/La4 : Gain  Gain=1/2  SaturateOnIntegerOverflow=on  OutDataTypeStr=Inherit: Same as input  ParamDataTypeStr=Inherit: Same as input
  Fcn : Fcn  Expr=((Ld+Ls)*u[1]+Ls*u[2]-(Ld+2*Ls)*u[3])/(2*Ld+3*Ls)
  Int : ResetIntegrator  InitialCondition=pi/3
  Log : Logic  Operator=NOT  Inputs=1
  Log1 : Logic
  Log2 : Logic  Operator=NOT  Inputs=1
  Log3 : Logic
  Log4 : Logic  Operator=NOT  Inputs=1
  Mux : Mux  Inputs=3
  Relay : Relay  OnSwitchValue=(2^.5)*Vph*sin(pi/6)  OffSwitchValue=0
  Sum : Sum  Inputs=-+  SaturateOnIntegerOverflow=on  InputSameDT=on  OutDataTypeStr=Inherit: Same as first input
  Sum3 : Sum  Inputs=-+-  SaturateOnIntegerOverflow=on  InputSameDT=on  OutDataTypeStr=Inherit: Same as first input
  Switch1 : Switch  Threshold=.5  SaturateOnIntegerOverflow=on  InputSameDT=on
  TETA : Constant  Value=100*pi
  comp : RelationalOperator  RndMeth=Nearest  InputSameDT=on
  logic2 : Logic  Operator=OR
  logic3 : Logic  Inputs=3
  logic4 : Logic  Operator=NOT  Inputs=1
  logic5 : Logic  Operator=OR
  logic7 : Logic  Inputs=3
  logic8 : Logic  Operator=OR
  mem{,1..4} (5 alike) : Memory
  mul : Product  SaturateOnIntegerOverflow=on  RndMeth=Zero  InputSameDT=on  OutDataTypeStr=Inherit: Same as first input
  mul1 : Product  SaturateOnIntegerOverflow=on  RndMeth=Zero  InputSameDT=on  OutDataTypeStr=Inherit: Same as first input
  out_2 : Outport
  out_1 : Outport  Port=2
  out_3 : Outport  Port=3
  out_4 : Outport  Port=4
  wires:
  comp/1 -> Log1/2, mem4/1
  mem4/1 -> mem/1
  mem/1 -> Log/1
  Sum/1 -> mul/2
  I4/1 -> Log3/1
  Switch1/1 -> out_2/1
  Log4/1 -> Switch1/2
  logic8/1 -> out_4/1, Log4/1, mem3/1, mul1/1
  mem3/1 -> Log3/2
  mul/1 -> Switch1/1
  Sum3/1 -> Switch1/3
  1/La3/1 -> Sum3/1
  1/La4/1 -> Sum3/3
  logic5/1 -> mul/1, mem2/1, logic7/2, out_1/1, mem1/1
  Log2/1 -> logic7/1
  di/1 -> logic3/2, logic7/3
  logic7/1 -> logic8/1
  Log3/1 -> logic8/2
  Log/1 -> Log1/1
  mem2/1 -> Log2/1
  logic3/1 -> logic5/1
  Relay/1 -> Int/2
  ot/1 -> logic4/1
  Te/1 -> comp/2
  Int/1 -> comp/1
  TETA/1 -> Int/1
  logic2/1 -> logic3/1
  0/1 -> Int/3
  Log1/1 -> logic5/2, logic2/2
  mem1/1 -> logic2/1
  logic4/1 -> logic3/3
  Mux/1 -> Fcn/1
  Fcn/1 -> mul1/2
  mul1/1 -> out_3/1
  vb/1 -> Relay/1, Sum/1, 1/La3/1, Mux/1
  vc/1 -> Sum/2, Sum3/2, Mux/2
  va/1 -> 1/La4/1, Mux/3

== system db4_8znzrb/Current-Controller with Current-sensor/I - Ctr/Adaptative Control ==
  Ia>0 : Inport
  Ia*- Iaf : Inport  Port=2
  3 : Constant  Value=0
  Gain : Gain  Gain=Kpi/TIi  SaturateOnIntegerOverflow=on  OutDataTypeStr=Inherit: Same as input  ParamDataTypeStr=Inherit: Same as input
  Gain1 : Gain  Gain=Kpi  SaturateOnIntegerOverflow=on  OutDataTypeStr=Inherit: Same as input  ParamDataTypeStr=Inherit: Same as input
  Gain2 : Gain  Gain=100*Kpi/TIi  SaturateOnIntegerOverflow=on  OutDataTypeStr=Inherit: Same as input  ParamDataTypeStr=Inherit: Same as input
  Limited Integrator : Integrator  LimitOutput=on  UpperSaturationLimit=VLL*sqrt(2)*3/pi  LowerSaturationLimit=-VLL*sqrt(2)*3/pi
  Sum : Sum  SaturateOnIntegerOverflow=on  InputSameDT=on  OutDataTypeStr=Inherit: Same as first input
  Switch : Switch  Threshold=.5  SaturateOnIntegerOverflow=on  InputSameDT=on
  Switch1 : Switch  Threshold=.5  SaturateOnIntegerOverflow=on  InputSameDT=on
  Vd* : Outport
  wires:
  Ia>0/1 -> Switch1/2, Switch/2
  3/1 -> Switch1/3
  Gain1/1 -> Switch1/1
  Gain2/1 -> Switch/3
  Switch/1 -> Limited Integrator/1
  Gain/1 -> Switch/1
  Ia*- Iaf/1 -> Gain2/1, Gain1/1, Gain/1
  Sum/1 -> Vd*/1
  Limited Integrator/1 -> Sum/1
  Switch1/1 -> Sum/2

== system db4_8znzrb/Permanent Magnet PMDCM/Converter with Zs 2 & 4 Quadrants/Subsystem ==
  In1 : Inport
  In2 : Inport  Port=2
  Gain1 : Gain  Gain=-1  SaturateOnIntegerOverflow=on  OutDataTypeStr=Inherit: Same as input  ParamDataTypeStr=Inherit: Same as input
  Switch3 : Switch  Threshold=.5  SaturateOnIntegerOverflow=on  InputSameDT=on
  Out1 : Outport
  wires:
  In2/1 -> Switch3/2
  Switch3/1 -> Out1/1
  In1/1 -> Gain1/1, Switch3/1
  Gain1/1 -> Switch3/3
